simulink library "WheelAssembly"  (R2015a)
settings: Solver=ode45  StartTime=0.0  StopTime=10.0  RelTol=1e-3
undefined symbols (not defined in the file): Motor
libraries: driveline x6, AMKMotor x3, simulink x1
settings Model: Creator=BRIAN  LastModifiedBy=tbria

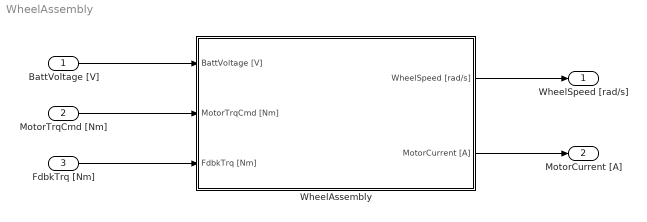
== system WheelAssembly ==
  BattVoltage [V] : Inport
  MotorTrqCmd [Nm] : Inport  Port=2
  FdbkTrq [Nm] : Inport  Port=3
  WheelAssembly : Subsystem
  WheelSpeed [rad/s] : Outport
  MotorCurrent [A] : Outport  Port=2
  wires:
  BattVoltage [V]/1 -> WheelAssembly/1(BattVoltage [V])
  MotorTrqCmd [Nm]/1 -> WheelAssembly/2(MotorTrqCmd [Nm])
  FdbkTrq [Nm]/1 -> WheelAssembly/3(FdbkTrq [Nm])
  WheelAssembly/1(WheelSpeed [rad/s]) -> WheelSpeed [rad/s]/1
  WheelAssembly/2(MotorCurrent [A]) -> MotorCurrent [A]/1

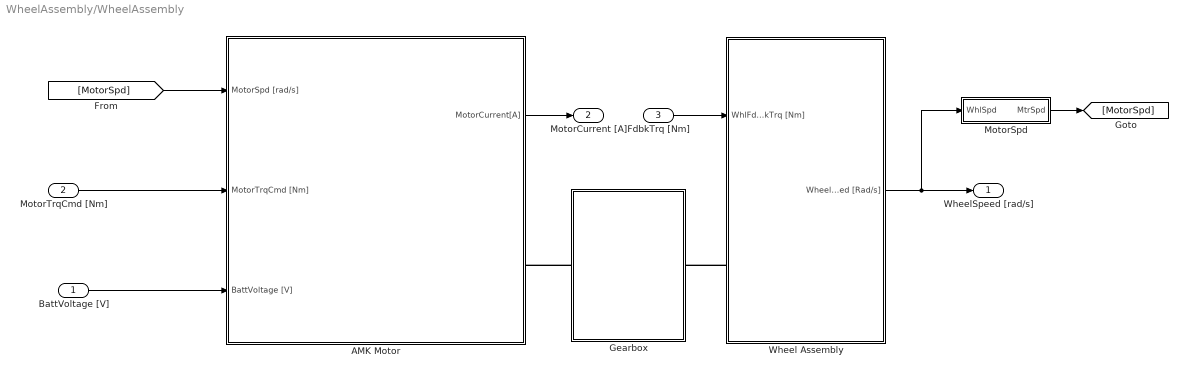
== system WheelAssembly/WheelAssembly ==
  BattVoltage [V] : Inport
  MotorTrqCmd [Nm] : Inport  Port=2
  FdbkTrq [Nm] : Inport  Port=3
  AMK Motor : Subsystem
  Gearbox : Subsystem
  MotorSpd : Subsystem
  Wheel Assembly : Subsystem
  WheelSpeed [rad/s] : Outport
  MotorCurrent [A] : Outport  Port=2
  wires:
  MotorTrqCmd [Nm]/1 -> AMK Motor/2(MotorTrqCmd [Nm])
  Wheel Assembly/1(WheelSpeed [Rad/s]) -> WheelSpeed [rad/s]/1, MotorSpd/1(WhlSpd)
  BattVoltage [V]/1 -> AMK Motor/3(BattVoltage [V])
  FdbkTrq [Nm]/1 -> Wheel Assembly/1(WhlFdbkTrq [Nm])
  [MotorSpd] -> AMK Motor/1(MotorSpd [rad/s])
  MotorSpd/1(MtrSpd) -> [MotorSpd]
  AMK Motor/1(MotorCurrent[A]) -> MotorCurrent [A]/1
  connections:
  Wheel Assembly/LConn1 -- Gearbox/RConn1
  Gearbox/LConn1 -- AMK Motor/RConn1

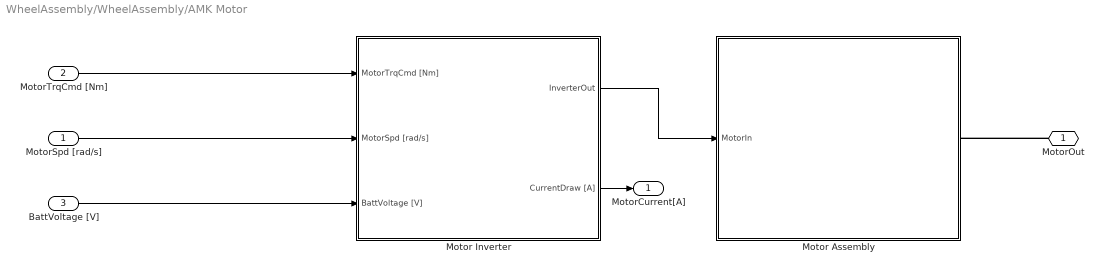
== system WheelAssembly/WheelAssembly/AMK Motor ==
  MotorSpd [rad/s] : Inport
  MotorTrqCmd [Nm] : Inport  Port=2
  BattVoltage [V] : Inport  Port=3
  Motor Assembly : Subsystem
  Motor Inverter : Subsystem
  MotorOut : PMIOPort  Port=1  Side=Right
  MotorCurrent[A] : Outport
  wires:
  BattVoltage [V]/1 -> Motor Inverter/3(BattVoltage [V])
  MotorSpd [rad/s]/1 -> Motor Inverter/2(MotorSpd [rad/s])
  MotorTrqCmd [Nm]/1 -> Motor Inverter/1(MotorTrqCmd [Nm])
  Motor Inverter/1(InverterOut) -> Motor Assembly/1(MotorIn)
  Motor Inverter/2(CurrentDraw [A]) -> MotorCurrent[A]/1
  connections:
  MotorOut/RConn1 -- Motor Assembly/RConn1

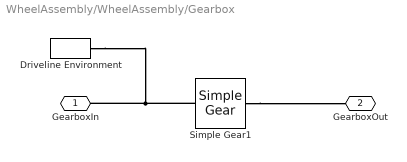
== system WheelAssembly/WheelAssembly/Gearbox ==
  Driveline Environment : driveline/Solver & Inertias/Driveline Environment  PortType=p1  BlockClass=Solver  PhysicalDomain=driveline_domain  SimulationMode=Dynamics  ModeIteration=on  DefaultClutchVelocityTolerance=1e-3  DefaultUseAutoClutchVelocityTolerance=off
  Simple Gear1 : driveline/Gears/Simple Gear  PortType=p1  BlockClass=SimpleGear  PhysicalDomain=driveline_domain  Reversing=off  Ratio=Motor.GR
  GearboxIn : PMIOPort  Port=1  Side=Left
  GearboxOut : PMIOPort  Port=2  Side=Right
  connections:
  Driveline Environment/LConn1 -- Simple Gear1/LConn1 -- GearboxIn/RConn1
  Simple Gear1/RConn1 -- GearboxOut/RConn1

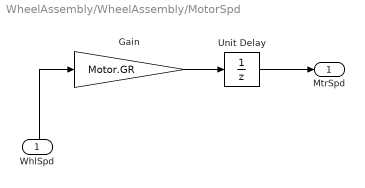
== system WheelAssembly/WheelAssembly/MotorSpd ==
  WhlSpd : Inport
  Gain : Gain  Gain=Motor.GR
  Unit Delay : UnitDelay  SampleTime=-1
  MtrSpd : Outport
  wires:
  Unit Delay/1 -> MtrSpd/1
  Gain/1 -> Unit Delay/1
  WhlSpd/1 -> Gain/1

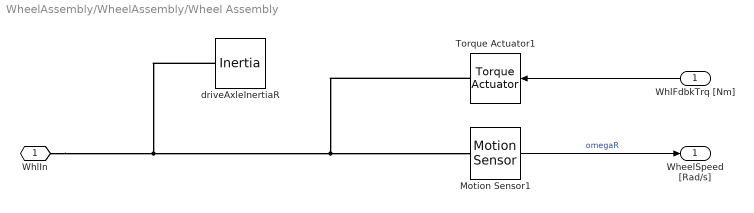
== system WheelAssembly/WheelAssembly/Wheel Assembly ==
  WhlFdbkTrq [Nm] : Inport
  Motion Sensor1 : driveline/Sensors & Actuators/Motion Sensor  Angle=off  x0=0  Velocity=on  Acceleration=off
  Torque Actuator1 : driveline/Sensors & Actuators/Torque Actuator
  driveAxleInertiaR : driveline/Solver & Inertias/Inertia  PortType=p1  BlockClass=Inertia  PhysicalDomain=driveline_domain  I=0.5  Ip=[]  Iv=[]  ShowLeft=on  ShowRight=off
  WhlIn : PMIOPort  Port=1  Side=Left
  WheelSpeed [Rad/s] : Outport
  wires:
  Motion Sensor1/1 -> WheelSpeed [Rad/s]/1  "omegaR"
  WhlFdbkTrq [Nm]/1 -> Torque Actuator1/1
  connections:
  WhlIn/RConn1 -- Motion Sensor1/LConn1 -- Torque Actuator1/RConn1 -- driveAxleInertiaR/LConn1

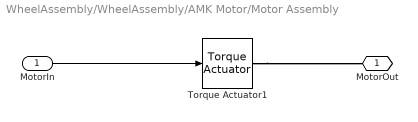
== system WheelAssembly/WheelAssembly/AMK Motor/Motor Assembly ==
  MotorIn : Inport
  Torque Actuator1 : driveline/Sensors & Actuators/Torque Actuator
  MotorOut : PMIOPort  Port=1  Side=Right
  wires:
  MotorIn/1 -> Torque Actuator1/1
  connections:
  Torque Actuator1/RConn1 -- MotorOut/RConn1

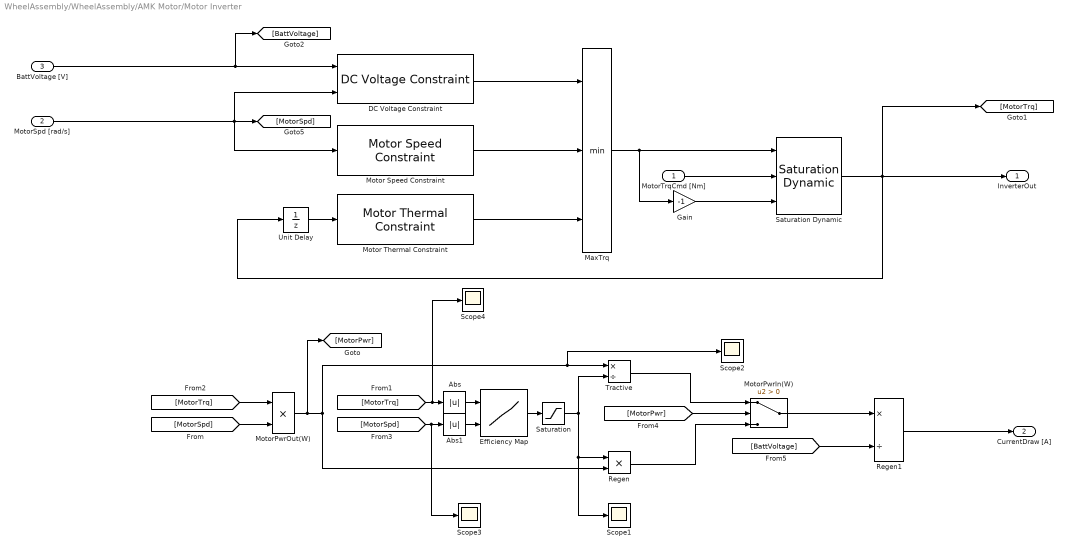
== system WheelAssembly/WheelAssembly/AMK Motor/Motor Inverter ==
  MotorTrqCmd [Nm] : Inport
  MotorSpd [rad/s] : Inport  Port=2
  BattVoltage [V] : Inport  Port=3
  Abs : Abs
  Abs1 : Abs
  DC Voltage Constraint : AMKMotor/WheelAssembly/AMK Motor/Motor Inverter/DC Voltage Constraint
  Efficiency Map : Lookup_n-D  BreakpointsForDimension1=Motor.Efficiency.Trq  BreakpointsForDimension2=Motor.Efficiency.Spd  Table=Motor.Efficiency.Eff  InternalRulePriority=Speed  RndMeth=Simplest  InputSameDT=on
  Gain : Gain  Gain=-1
  MaxTrq : MinMax  Inputs=3
  Motor Speed Constraint : AMKMotor/WheelAssembly/AMK Motor/Motor Inverter/Motor Speed Constraint
  Motor Thermal Constraint : AMKMotor/WheelAssembly/AMK Motor/Motor Inverter/Motor Thermal Constraint
  MotorPwrIn(W) : Switch  Criteria=u2 > Threshold
  MotorPwrOut(W) : Product
  Regen : Product
  Regen1 : Product  Inputs=*/
  Saturation : Saturate  UpperLimit=1  LowerLimit=0
  Saturation Dynamic : simulink/Discontinuities/Saturation Dynamic  OutMin=[]  OutMax=[]  OutDataTypeStr=Inherit: Same as second input  OutDataType=fixdt(1, 16)  OutScaling=2^-10  DoSatur=off
  Scope{1..4} (4 alike) : Scope
      Scope1 settings: YMin=0  YMax=1  SaveName=ScopeData16
      Scope2 settings: YMin=-0  YMax=18000  SaveName=ScopeData17
      Scope3 settings: YMin=0  YMax=21  SaveName=ScopeData18
      Scope4 settings: YMin=0  YMax=21  SaveName=ScopeData19
  Tractive : Product  Inputs=*/
  Unit Delay : UnitDelay  SampleTime=-1
  InverterOut : Outport
  CurrentDraw [A] : Outport  Port=2
  wires:
  MotorTrqCmd [Nm]/1 -> Saturation Dynamic/2
  DC Voltage Constraint/1 -> MaxTrq/1
  Motor Speed Constraint/1 -> MaxTrq/2
  Motor Thermal Constraint/1 -> MaxTrq/3
  Gain/1 -> Saturation Dynamic/3
  Unit Delay/1 -> Motor Thermal Constraint/1
  Saturation Dynamic/1 -> [MotorTrq], Unit Delay/1, InverterOut/1
  MaxTrq/1 -> Saturation Dynamic/1, Gain/1
  MotorSpd [rad/s]/1 -> DC Voltage Constraint/2, Motor Speed Constraint/1, [MotorSpd]
  [MotorSpd] -> MotorPwrOut(W)/2
  [MotorTrq] -> Scope4/1, Abs/1
  [MotorTrq] -> MotorPwrOut(W)/1
  [MotorSpd] -> Scope3/1, Abs1/1
  [MotorPwr] -> MotorPwrIn(W)/2
  MotorPwrOut(W)/1 -> [MotorPwr], Regen/2, Scope2/1, Tractive/1
  Efficiency Map/1 -> Saturation/1
  Tractive/1 -> MotorPwrIn(W)/1
  Regen/1 -> MotorPwrIn(W)/3
  BattVoltage [V]/1 -> [BattVoltage], DC Voltage Constraint/1
  MotorPwrIn(W)/1 -> Regen1/1
  [BattVoltage] -> Regen1/2
  Regen1/1 -> CurrentDraw [A]/1
  Saturation/1 -> Scope1/1, Regen/1, Tractive/2
  Abs/1 -> Efficiency Map/1
  Abs1/1 -> Efficiency Map/2
